simulink model "Rotary_Inverted_Pendulum_HIL_Tutorial_R2018"  (R2018a)
settings: Solver=FixedStepAuto  StartTime=0.0  StopTime=inf  RelTol=1e-3  EnableMultiTasking=on
undefined symbols (not defined in the file): k
libraries: arduinolib x3, simulink_extras x2
settings Model: SimulationMode=external  ExtModeTrigDuration=2  Creator=hima_  LastModifiedBy=Ahmed
settings DataIOCC: ReturnWorkspaceOutputs=on
settings OptimizationCC: EnhancedBackFolding=on  PassReuseOutputArgsAs=Individual arguments  ZeroExternalMemoryAtStartup=off  ZeroInternalMemoryAtStartup=off  MaxStackSize=64  OptimizeBlockOrder=speed  DifferentSizesBufferReuse=on  OptimizationCustomize=off
settings DebuggingCC: ParameterTunabilityLossMsg=error
settings HardwareCC: ProdBitPerInt=16  ProdBitPerPointer=16  ProdBitPerSizeT=16  ProdBitPerPtrDiffT=16  ProdLargestAtomicFloat=None  ProdWordSize=8  ProdHWDeviceType=Atmel->AVR
settings SFSimCC: SimUseLocalCustomCode=on  MATLABDynamicMemAlloc=off
settings RTWCC: SystemTargetFile=ert.tlc  HardwareBoard=Arduino Mega 2560  TLCOptions=-aInlineSetEventsForThisBaseRateFcn=TLC_FALSE -aSuppressMultiTaskScheduler=TLC_FALSE -aRateBasedStepFcn=1  TemplateMakefile=ert_default_tmf  RTWUseLocalCustomCode=on  Toolchain=Arduino AVR  BuildConfiguration=Faster Runs
settings CodeAppCC: ForceParamTrailComments=on  IgnoreCustomStorageClasses=off  OperatorAnnotations=on  SimulinkDataObjDesc=on  SFDataObjDesc=on  InsertBlockDesc=on
settings ERTTargetCC: SupportContinuousTime=on  SupportVariableSizeSignals=on  ExtModeTransport=3  ExtModeStaticAlloc=on  ExtModeStaticAllocSize=2048  ExtModeMexFile=ext_xcp  ExtModeIntrfLevel=Level2 - Open

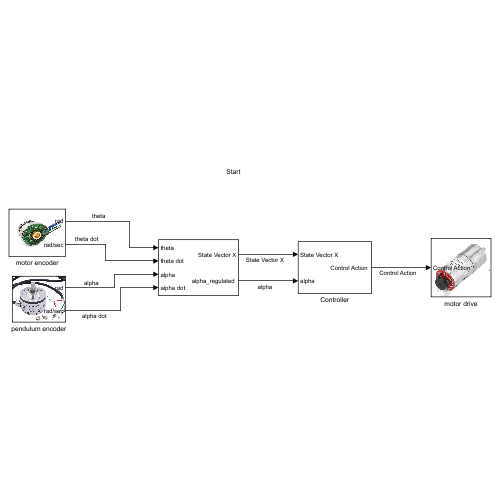
[thumbnail: Simulink's stored preview of the top-level diagram]
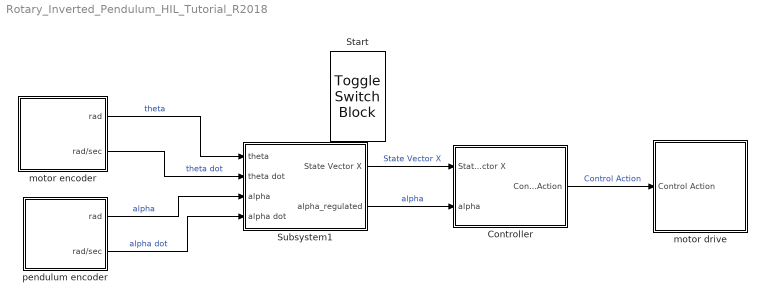
== system Rotary_Inverted_Pendulum_HIL_Tutorial_R2018 ==
  Controller : Subsystem
  Start : ToggleSwitchBlock  LabelPosition=Hide  WebBlockId=55
      settings: Values={{'Off', 'On'}, [0 1]}
  Subsystem1 : Subsystem
  motor drive : Subsystem
      mask Display: image('Screenshot2022_12_23124832.png'); % Use "Edit Image" on toolstrip to change.
  motor encoder : Subsystem
      mask Display: image('motorEncoder.jpg');
  pendulum encoder : Subsystem
      mask Display: image('encoder.jpg');
  wires:
  motor encoder/1(rad) -> Subsystem1/1(theta)  "theta"
  motor encoder/2(rad/sec) -> Subsystem1/2(theta dot)  "theta dot"
  pendulum encoder/1(rad) -> Subsystem1/3(alpha)  "alpha"
  pendulum encoder/2(rad/sec) -> Subsystem1/4(alpha dot)  "alpha dot"
  Subsystem1/1(State Vector X) -> Controller/1(State Vector X)  "State Vector X"
  Subsystem1/2("alpha_regulated ") -> Controller/2(alpha)  "alpha"
  Controller/1("Control Action ") -> motor drive/1(Control Action)  "Control Action"

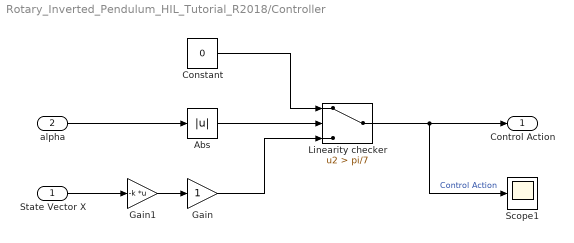
== system Rotary_Inverted_Pendulum_HIL_Tutorial_R2018/Controller ==
  State Vector X : Inport
  alpha : Inport  Port=2
  Abs : Abs
  Constant : Constant  Value=0
  Gain : Gain
  Gain1 : Gain  Gain=-k  Multiplication=Matrix(K*u)
  Linearity checker : Switch  Criteria=u2 > Threshold  Threshold=pi/7
  Scope1 : Scope
  "Control Action " : Outport
  wires:
  State Vector X/1 -> Gain1/1
  Constant/1 -> Linearity checker/1
  Linearity checker/1 -> "Control Action "/1, Scope1/1  "Control Action"
  Gain1/1 -> Gain/1
  Gain/1 -> Linearity checker/3
  Abs/1 -> Linearity checker/2
  alpha/1 -> Abs/1

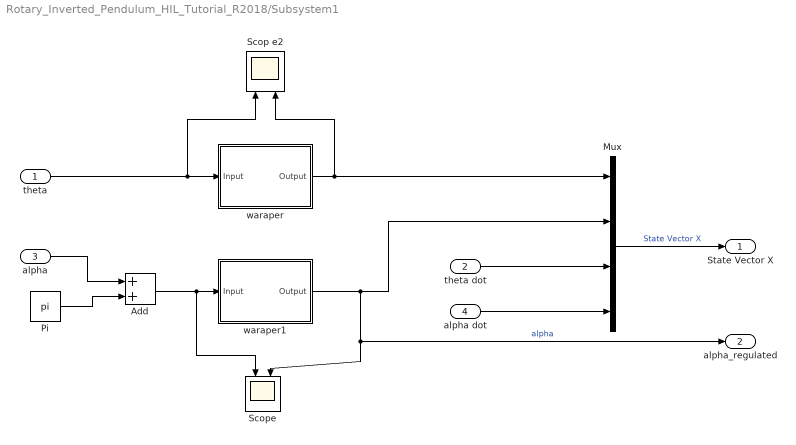
== system Rotary_Inverted_Pendulum_HIL_Tutorial_R2018/Subsystem1 ==
  theta : Inport
  theta dot : Inport  Port=2
  alpha : Inport  Port=3
  alpha dot : Inport  Port=4
  Add : Sum
  Mux : Mux
  Pi : Constant  Value=pi  OutDataTypeStr=Inherit: Inherit via back propagation
  Scop e2 : Scope  NumInputPorts=2
  Scope : Scope  NumInputPorts=2
  waraper : Subsystem
  waraper1 : Subsystem
  State Vector X : Outport
  "alpha_regulated " : Outport  Port=2
  wires:
  theta/1 -> Scop e2/1, waraper/1(Input)
  Mux/1 -> State Vector X/1  "State Vector X"
  waraper/1(Output) -> Mux/1, Scop e2/2
  alpha dot/1 -> Mux/4
  Pi/1 -> Add/2
  Add/1 -> Scope/1, waraper1/1(Input)
  waraper1/1(Output) -> Mux/2, "alpha_regulated "/1, Scope/2  "alpha"
  alpha/1 -> Add/1
  theta dot/1 -> Mux/3

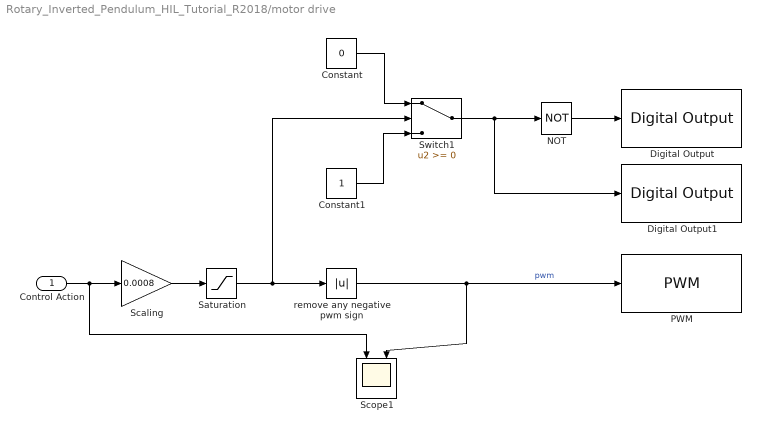
== system Rotary_Inverted_Pendulum_HIL_Tutorial_R2018/motor drive ==
  Control Action : Inport
  Constant : Constant  Value=0
  Constant1 : Constant
  Digital Output : arduinolib/Digital Output  pinNumber=7  Direction=output  blockPlatform=arduino
  Digital Output1 : arduinolib/Digital Output  pinNumber=8  Direction=output  blockPlatform=arduino
  NOT : Logic  Operator=NOT  IconShape=distinctive  AllPortsSameDT=off  OutDataTypeStr=boolean
  PWM : arduinolib/PWM  pinNumber=6  frequencyType=Default  desiredFrequency=490.2  achievableFrequency=490.2
  Saturation : Saturate  UpperLimit=255  LowerLimit=-255
  Scaling : Gain  Gain=0.0008
  Scope1 : Scope  NumInputPorts=2
  Switch1 : Switch
  remove any negative pwm sign : Abs
  wires:
  remove any negative pwm sign/1 -> PWM/1, Scope1/2  "pwm"
  Saturation/1 -> Switch1/2, remove any negative pwm sign/1
  Constant/1 -> Switch1/1
  NOT/1 -> Digital Output/1
  Switch1/1 -> Digital Output1/1, NOT/1
  Control Action/1 -> Scope1/1, Scaling/1
  Scaling/1 -> Saturation/1
  Constant1/1 -> Switch1/3

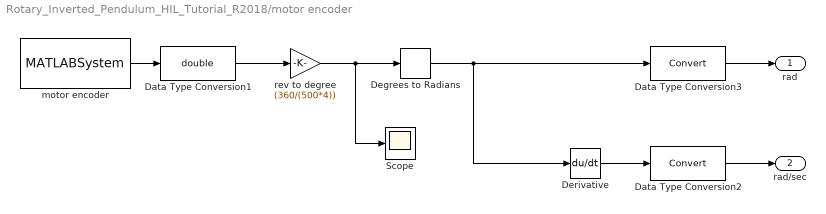
== system Rotary_Inverted_Pendulum_HIL_Tutorial_R2018/motor encoder ==
  Data Type Conversion1 : DataTypeConversion  OutDataTypeStr=double
  Data Type Conversion2 : DataTypeConversion
  Data Type Conversion3 : DataTypeConversion
  Degrees to Radians : simulink_extras/Transformations/Degrees to Radians
  Derivative : Derivative
  Scope : Scope
  motor encoder : MATLABSystem  System=Encoder_arduino  Encoder=1  PinA=18  PinB=19  SampleTime=0.001
      mask Type: Encoder_arduino
      mask Display:
      | disp('Encoder');
      | port_label('output',1,'y');
  rev to degree : Gain  Gain=(360/(500*4))
  rad : Outport
  rad/sec : Outport  Port=2
  wires:
  Derivative/1 -> Data Type Conversion2/1
  rev to degree/1 -> Scope/1, Degrees to Radians/1
  Degrees to Radians/1 -> Derivative/1, Data Type Conversion3/1
  Data Type Conversion3/1 -> rad/1
  Data Type Conversion2/1 -> rad/sec/1
  Data Type Conversion1/1 -> rev to degree/1
  motor encoder/1 -> Data Type Conversion1/1

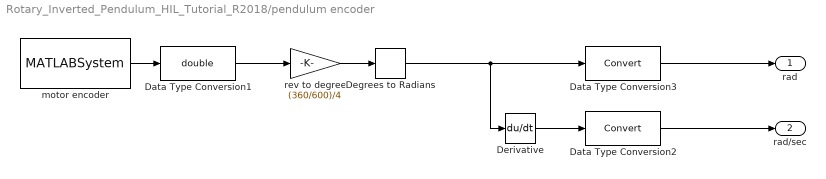
== system Rotary_Inverted_Pendulum_HIL_Tutorial_R2018/pendulum encoder ==
  Data Type Conversion1 : DataTypeConversion  OutDataTypeStr=double
  Data Type Conversion2 : DataTypeConversion
  Data Type Conversion3 : DataTypeConversion
  Degrees to Radians : simulink_extras/Transformations/Degrees to Radians
  Derivative : Derivative
  motor encoder : MATLABSystem  System=Encoder_arduino  Encoder=0  PinA=2  PinB=3  SampleTime=0.001
      mask Type: Encoder_arduino
      mask Display:
      | disp('Encoder');
      | port_label('output',1,'y');
  rev to degree : Gain  Gain=(360/600)/4
  rad : Outport
  rad/sec : Outport  Port=2
  wires:
  motor encoder/1 -> Data Type Conversion1/1
  Data Type Conversion3/1 -> rad/1
  Data Type Conversion2/1 -> rad/sec/1
  Data Type Conversion1/1 -> rev to degree/1
  rev to degree/1 -> Degrees to Radians/1
  Degrees to Radians/1 -> Derivative/1, Data Type Conversion3/1
  Derivative/1 -> Data Type Conversion2/1

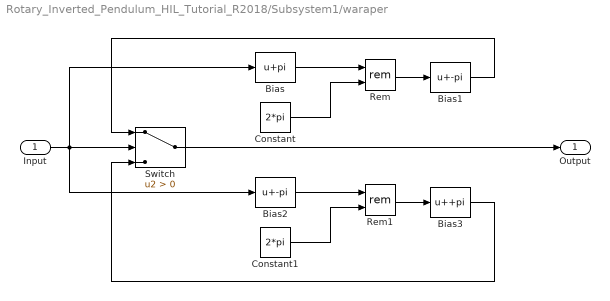
== system Rotary_Inverted_Pendulum_HIL_Tutorial_R2018/Subsystem1/waraper ==
  Input : Inport
  Bias : Bias  Bias=pi
  Bias1 : Bias  Bias=-pi
  Bias2 : Bias  Bias=-pi
  Bias3 : Bias  Bias=+pi
  Constant : Constant  Value=2*pi
  Constant1 : Constant  Value=2*pi
  Rem : Math  Operator=rem  SaturateOnIntegerOverflow=on
  Rem1 : Math  Operator=rem  SaturateOnIntegerOverflow=on
  Switch : Switch  Criteria=u2 > Threshold
  Output : Outport
  wires:
  Constant/1 -> Rem/2
  Bias/1 -> Rem/1
  Input/1 -> Bias/1, Bias2/1, Switch/2
  Bias3/1 -> Switch/3
  Bias2/1 -> Rem1/1
  Rem1/1 -> Bias3/1
  Constant1/1 -> Rem1/2
  Switch/1 -> Output/1
  Rem/1 -> Bias1/1
  Bias1/1 -> Switch/1

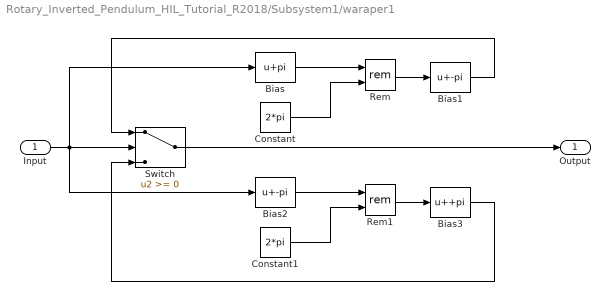
== system Rotary_Inverted_Pendulum_HIL_Tutorial_R2018/Subsystem1/waraper1 ==
  Input : Inport
  Bias : Bias  Bias=pi
  Bias1 : Bias  Bias=-pi
  Bias2 : Bias  Bias=-pi
  Bias3 : Bias  Bias=+pi
  Constant : Constant  Value=2*pi
  Constant1 : Constant  Value=2*pi
  Rem : Math  Operator=rem  SaturateOnIntegerOverflow=on
  Rem1 : Math  Operator=rem  SaturateOnIntegerOverflow=on
  Switch : Switch
  Output : Outport
  wires:
  Constant/1 -> Rem/2
  Bias/1 -> Rem/1
  Input/1 -> Bias/1, Bias2/1, Switch/2
  Bias3/1 -> Switch/3
  Bias2/1 -> Rem1/1
  Rem1/1 -> Bias3/1
  Constant1/1 -> Rem1/2
  Switch/1 -> Output/1
  Rem/1 -> Bias1/1
  Bias1/1 -> Switch/1
